simulink subsystem "L2"  (R2024a)
settings: Solver=VariableStepAuto  StartTime=0.0  StopTime=10.0  RelTol=1e-3
undefined symbols (not defined in the file or in its folder): D, r
libraries: inductance x1
settings Model: Creator=Bocchio  LastModifiedBy=Bocchio

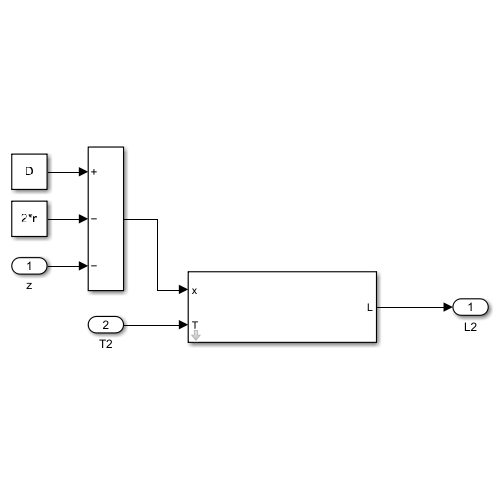
[thumbnail: Simulink's stored preview of the top-level diagram]
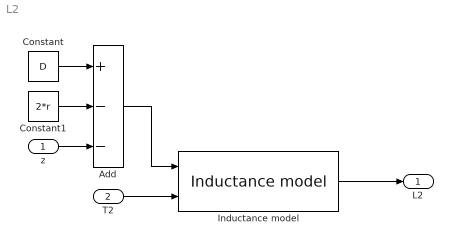
== system L2 ==
  z : Inport
  T2 : Inport  Port=2
  Add : Sum  Inputs=+--
  Constant : Constant  Value=D
  Constant1 : Constant  Value=2*r
  Inductance model : inductance/Inductance model  L0=L20  Lx=L2x  a=a
  L2 : Outport
  wires:
  Inductance model/1 -> L2/1
  T2/1 -> Inductance model/2
  z/1 -> Add/3
  Add/1 -> Inductance model/1
  Constant/1 -> Add/1
  Constant1/1 -> Add/2
